simulink model "no_oss"  (R2024b)
settings: Solver=VariableStepAuto  StartTime=0.0  StopTime=100  RelTol=1e-3
values from neighbouring files (symbols this model uses):
  A4 = horzcat([0;0;0;0], A4)    [stabilita_AS.m]
  BB = [0; B]    [stabilita_AS.m]
  C = [1 0 0 0 ... (first row only)    [stabilita_AS.m]
  KK = [0 K]    [stabilita_AS.m]
  L_oss = (1/epsilon) * L0    [stabilita_AS.m]
undefined symbols (not defined in the file or in its folder): L_oss_theta
settings Model: Creator=costa  LastModifiedBy=costa

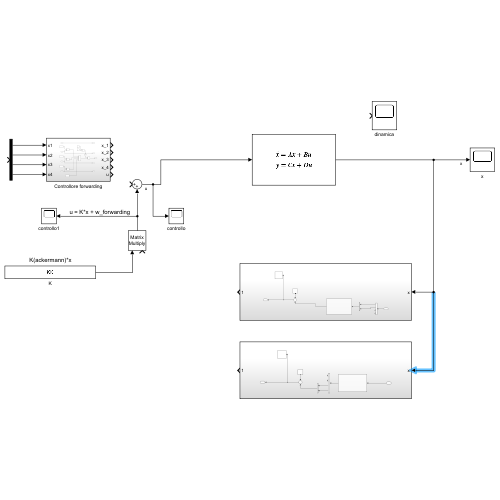
[thumbnail: Simulink's stored preview of the top-level diagram]
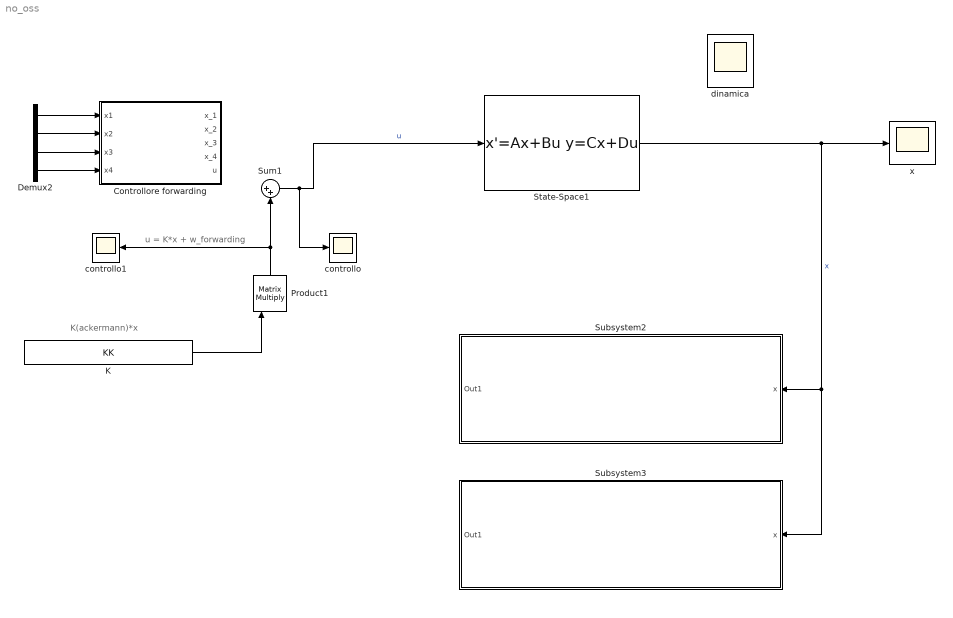
== system no_oss ==
  note: u = K*x + w_forwarding
  note: K(ackermann)*x
  Controllore forwarding : Subsystem
  Demux2 : Demux
  K : Constant  Value=KK  VectorParams1D=off
  Product1 : Product  Multiplication=Matrix(*)
  State-Space1 : StateSpace  A=A4  B=BB  C=eye(4)  D=[0; 0; 0; 0]  InitialCondition=0
  Subsystem2 : Subsystem
  Subsystem3 : Subsystem
  Sum1 : Sum  Inputs=|++
  controllo : Scope
  controllo1 : Scope
  dinamica : Scope
  x : Scope
  wires:
  Demux2/2 -> Controllore forwarding/2(x2)
  Demux2/3 -> Controllore forwarding/3(x3)
  Demux2/4 -> Controllore forwarding/4(x4)
  Product1/1 -> controllo1/1, Sum1/2
  K/1 -> Product1/1
  Sum1/1 -> State-Space1/1, controllo/1  "u"
  State-Space1/1 -> Subsystem2/1(x), Subsystem3/1(x), x/1  "x"
  Demux2/1 -> Controllore forwarding/1(x1)

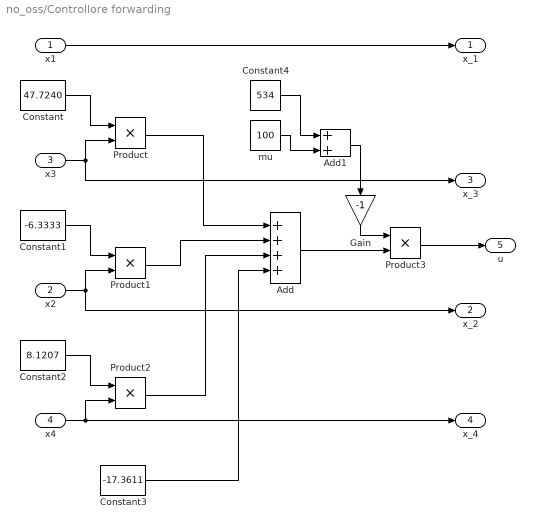
== system no_oss/Controllore forwarding ==
  x1 : Inport
  x2 : Inport  Port=2
  x3 : Inport  Port=3
  x4 : Inport  Port=4
  Add : Sum  Inputs=++++
  Add1 : Sum
  Constant : Constant  Value=47.7240
  Constant1 : Constant  Value=-6.3333
  Constant2 : Constant  Value=8.1207
  Constant3 : Constant  Value=-17.3611
  Constant4 : Constant  Value=534
  Gain : Gain  Gain=-1
  Product{,1..3} (4 alike) : Product
  mu : Constant  Value=100
  x_1 : Outport
  x_2 : Outport  Port=2
  x_3 : Outport  Port=3
  x_4 : Outport  Port=4
  u : Outport  Port=5
  wires:
  x3/1 -> x_3/1, Product/2
  Constant/1 -> Product/1
  Constant1/1 -> Product1/1
  x2/1 -> Product1/2, x_2/1
  Constant2/1 -> Product2/1
  x4/1 -> x_4/1, Product2/2
  Product/1 -> Add/1
  Product1/1 -> Add/2
  Product2/1 -> Add/3
  Constant3/1 -> Add/4
  Add/1 -> Product3/2
  Product3/1 -> u/1
  x1/1 -> x_1/1
  Constant4/1 -> Add1/1
  mu/1 -> Add1/2
  Add1/1 -> Gain/1
  Gain/1 -> Product3/1

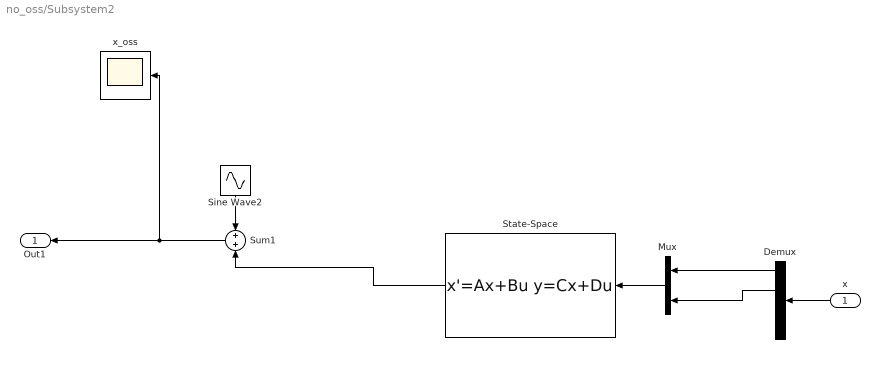
== system no_oss/Subsystem2 ==
  x : Inport
  Demux : Demux
  Mux : Mux  Inputs=2
  Sine Wave2 : Sin  Amplitude=0.1  Frequency=2*pi*50  SampleTime=0
  State-Space : StateSpace  A=A4-L_oss*C  B=L_oss  C=[1 0 0 0; 0 1 0 0]  D=[0 0; 0 0]  InitialCondition=0  AbsoluteTolerance=1e-4
  Sum1 : Sum
  x_oss : Scope
  Out1 : Outport
  wires:
  State-Space/1 -> Sum1/2
  x/1 -> Demux/1
  Demux/1 -> Mux/1
  Demux/2 -> Mux/2
  Sine Wave2/1 -> Sum1/1
  Sum1/1 -> x_oss/1, Out1/1
  Mux/1 -> State-Space/1

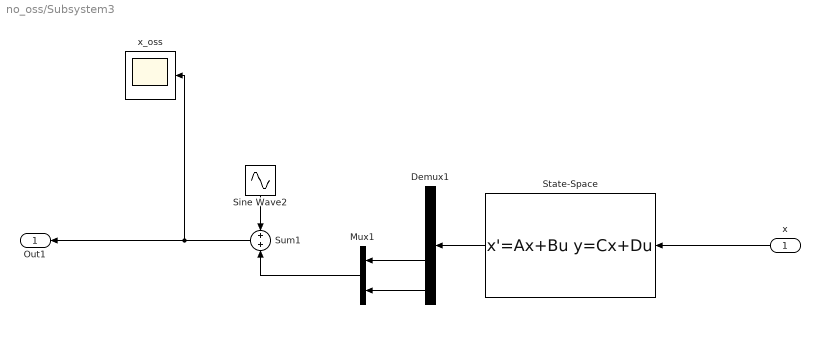
== system no_oss/Subsystem3 ==
  x : Inport
  Demux1 : Demux
  Mux1 : Mux  Inputs=2
  Sine Wave2 : Sin  Amplitude=0.1  Frequency=2*pi*50  SampleTime=0
  State-Space : StateSpace  A=A4-L_oss_theta*eye(4)  B=L_oss_theta  C=eye(4)  D=[0 0 0 0;0 0 0 0; 0 0 0 0; 0 0 0 0]  InitialCondition=[1 2 0 1]  AbsoluteTolerance=1e-4
  Sum1 : Sum
  x_oss : Scope
  Out1 : Outport
  wires:
  Sine Wave2/1 -> Sum1/1
  Sum1/1 -> x_oss/1, Out1/1
  State-Space/1 -> Demux1/1
  Demux1/3 -> Mux1/1
  Demux1/4 -> Mux1/2
  Mux1/1 -> Sum1/2
  x/1 -> State-Space/1
